simulink model "recursive_running_sum_single"  (R2014b)
settings: Solver=ode45  StartTime=0.0  StopTime=inf  RelTol=1e-3
undefined symbols (not defined in the file or in its folder): filtk
settings Model: Creator=Ben  LastModifiedBy=Ben

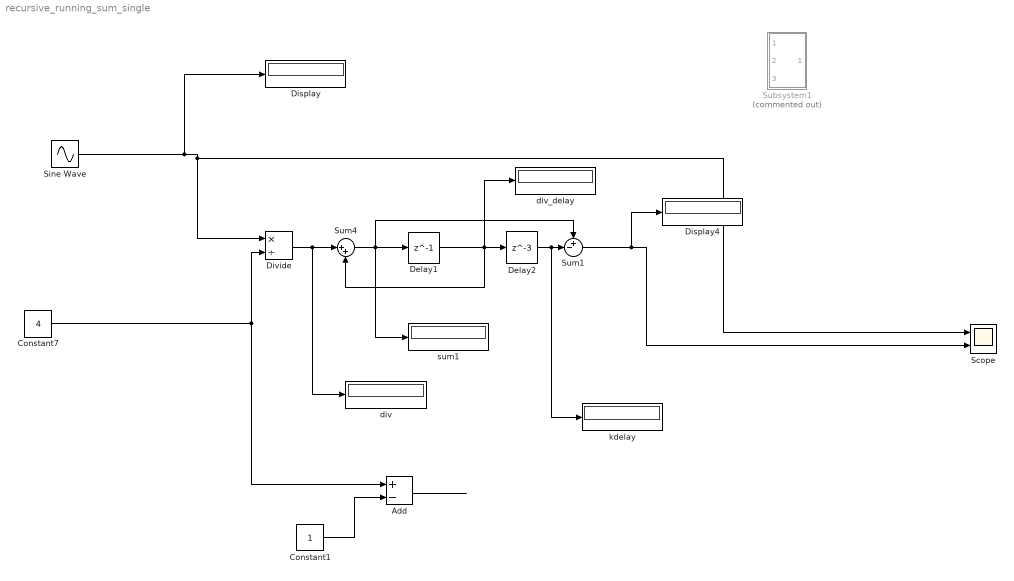
== system recursive_running_sum_single ==
  Add : Sum  Inputs=+-
  Constant1 : Constant
  Constant7 : Constant  Value=4
  Delay1 : Delay  DelayLength=1  InitialCondition=0
  Delay2 : Delay  DelayLength=3  InitialCondition=0
  Display : Display
  Display4 : Display
  Divide : Product  Inputs=*/
  Scope : Scope  NumInputPorts=2
      settings: TimeRange=0.0001  YMin=-1~-1  YMax=1~1
  Sine Wave : Sin  Frequency=1E6*2*pi  SampleTime=1/250E6
  Subsystem1 : Subsystem  Commented=on
  Sum1 : Sum  Inputs=+-|
  Sum4 : Sum  Inputs=|++
  div : Display
  div_delay : Display
  "kdelay " : Display
  sum1 : Display
  wires:
  Sum1/1 -> Display4/1, Scope/2
  Constant7/1 -> Add/1, Divide/2
  Add/1 -> ?
  Divide/1 -> div/1, Sum4/1
  Delay2/1 -> "kdelay "/1, Sum1/2
  Delay1/1 -> div_delay/1, Sum4/2, Delay2/1
  Sum4/1 -> sum1/1, Sum1/1, Delay1/1
  Constant1/1 -> Add/2
  Sine Wave/1 -> Display/1, Scope/1, Divide/1

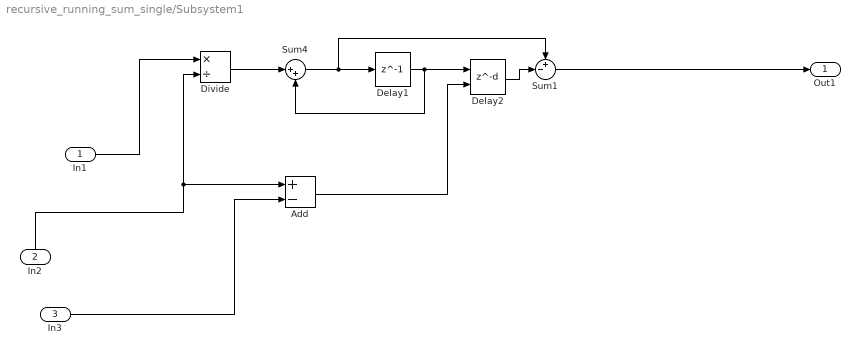
== system recursive_running_sum_single/Subsystem1 ==
  In1 : Inport
  In2 : Inport  Port=2
  In3 : Inport  Port=3
  Add : Sum  Inputs=+-
  Delay1 : Delay  DelayLength=1  InitialCondition=0
  Delay2 : Delay  DelayLengthSource=Input port  DelayLength=filtk-1  InitialCondition=0
      settings: InputPortMap=u0,p1
  Divide : Product  Inputs=*/
  Sum1 : Sum  Inputs=+-|
  Sum4 : Sum  Inputs=|++
  Out1 : Outport
  wires:
  Sum4/1 -> Sum1/1, Delay1/1
  Delay1/1 -> Delay2/1, Sum4/2
  Delay2/1 -> Sum1/2
  Sum1/1 -> Out1/1
  In1/1 -> Divide/1
  Divide/1 -> Sum4/1
  Add/1 -> Delay2/2
  In2/1 -> Divide/2, Add/1
  In3/1 -> Add/2
